simulink model "MassTransfer"  (R2023a)
settings: Solver=ode4  StartTime=0.0  StopTime=7540  FixedStep=Delta  RelTol=1e-3
values from neighbouring files (symbols this model uses):
  C2Ini = 1.6    [MassTransferModelData.m]
  C3Ini = 0    [MassTransferModelData.m]
  C4Ini = 0    [MassTransferModelData.m]
  C5Ini = 1.6    [MassTransferModelData.m]
  Delta = 5    [MassTransferModelData.m]
  F = 96485    [MassTransferModelData.m]
  NCells = 120    [MassTransferModelData.m]
  VCell = 0.4968    [MassTransferModelData.m]
  VTank = 500    [MassTransferModelData.m]
  z = 1    [MassTransferModelData.m]
undefined symbols (not defined in the file or in its folder): DiscIntNeverNeededParam
(part 1 of 3)
settings Model: Creator=801896  LastModifiedBy=801896

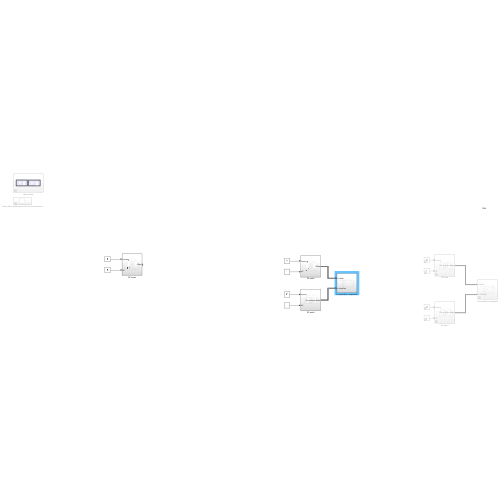
[thumbnail: Simulink's stored preview of the top-level diagram]
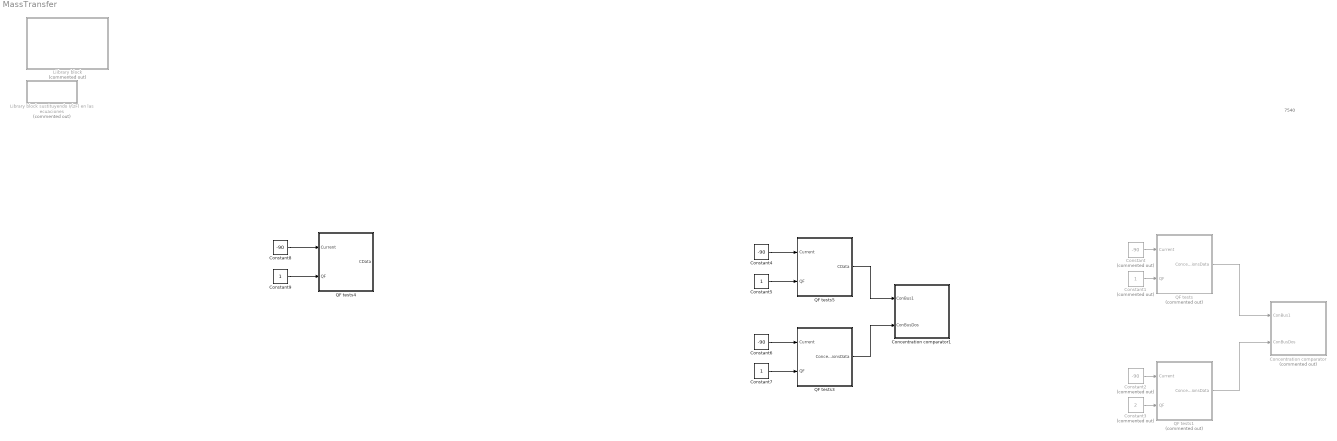
== system MassTransfer ==
  note: 7540
  Concentration comparator : Subsystem  Commented=on
  Concentration comparator1 : Subsystem
  Constant : Constant  Commented=on  Value=-90
  Constant1 : Constant  Commented=on
  Constant2 : Constant  Commented=on  Value=-90
  Constant3 : Constant  Commented=on  Value=2
  Constant4 : Constant  Value=-90
  Constant5 : Constant
  Constant6 : Constant  Value=-90
  Constant7 : Constant
  Constant8 : Constant  Value=-90
  Constant9 : Constant
  Library block sustituyendo I/(zF) en las ecuaciones : Subsystem  Commented=on
  Liibrary block : Subsystem  Commented=on
  QF tests : Subsystem  Commented=on
  QF tests1 : Subsystem  Commented=on
  QF tests3 : Subsystem
  QF tests4 : Subsystem
  QF tests5 : Subsystem
  wires:
  Constant/1 -> QF tests/1(Current)
  Constant1/1 -> QF tests/2(QF)
  Constant2/1 -> QF tests1/1(Current)
  Constant3/1 -> QF tests1/2(QF)
  QF tests/1(ConcentrationsData) -> Concentration comparator/1(ConBus1)
  QF tests1/1(ConcentrationsData) -> Concentration comparator/2(ConBusDos)
  Constant4/1 -> QF tests5/1(Current)
  Constant5/1 -> QF tests5/2(QF)
  Constant6/1 -> QF tests3/1(Current)
  Constant7/1 -> QF tests3/2(QF)
  QF tests5/1(CData) -> Concentration comparator1/1(ConBus1)
  QF tests3/1(ConcentrationsData) -> Concentration comparator1/2(ConBusDos)
  Constant8/1 -> QF tests4/1(Current)
  Constant9/1 -> QF tests4/2(QF)

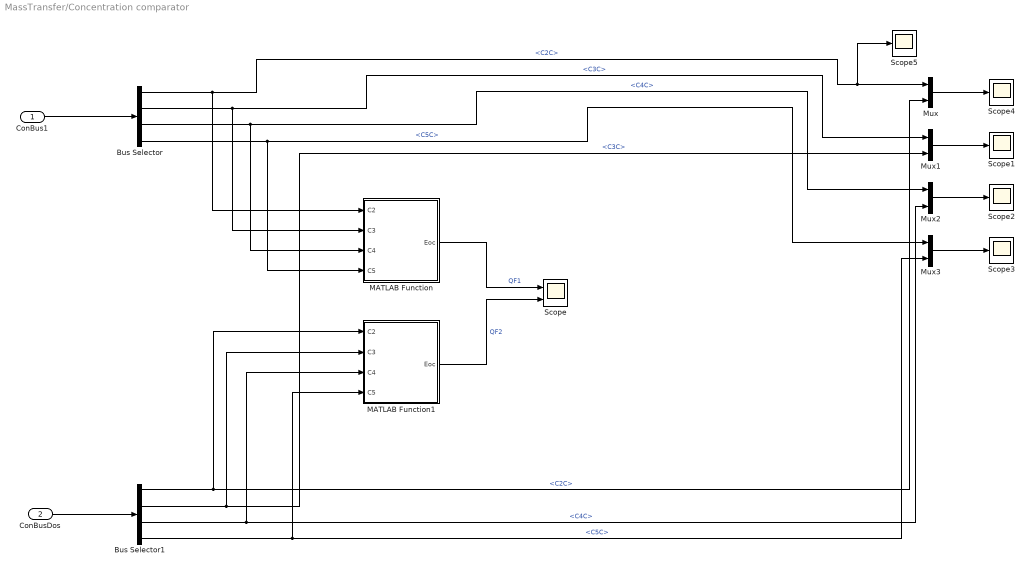
== system MassTransfer/Concentration comparator ==
  ConBus1 : Inport
  ConBusDos : Inport  Port=2
  Bus Selector : BusSelector  OutputSignals=C2C,C3C,C4C,C5C
  Bus Selector1 : BusSelector  OutputSignals=C2C,C3C,C4C,C5C
  MATLAB Function : MATLAB Function  TreatAsAtomicUnit=on
  MATLAB Function1 : MATLAB Function  TreatAsAtomicUnit=on
  Mux{,1..3} (4 alike) : Mux  Inputs=2
  Scope : Scope  NumInputPorts=2
  Scope{1..5} (5 alike) : Scope
  wires:
  ConBus1/1 -> Bus Selector/1
  ConBusDos/1 -> Bus Selector1/1
  Bus Selector/1 -> MATLAB Function/1(C2), Scope5/1, Mux/1  "<C2C>"
  Bus Selector1/1 -> MATLAB Function1/1(C2), Mux/2  "<C2C>"
  Bus Selector/2 -> MATLAB Function/2(C3), Mux1/1  "<C3C>"
  Bus Selector1/2 -> MATLAB Function1/2(C3), Mux1/2  "<C3C>"
  Bus Selector/3 -> MATLAB Function/3(C4), Mux2/1  "<C4C>"
  Bus Selector1/3 -> MATLAB Function1/3(C4), Mux2/2  "<C4C>"
  Bus Selector1/4 -> MATLAB Function1/4(C5), Mux3/2  "<C5C>"
  Bus Selector/4 -> MATLAB Function/4(C5), Mux3/1  "<C5C>"
  Mux1/1 -> Scope1/1
  Mux2/1 -> Scope2/1
  Mux3/1 -> Scope3/1
  Mux/1 -> Scope4/1
  MATLAB Function/1(Eoc) -> Scope/1  "QF1"
  MATLAB Function1/1(Eoc) -> Scope/2  "QF2"

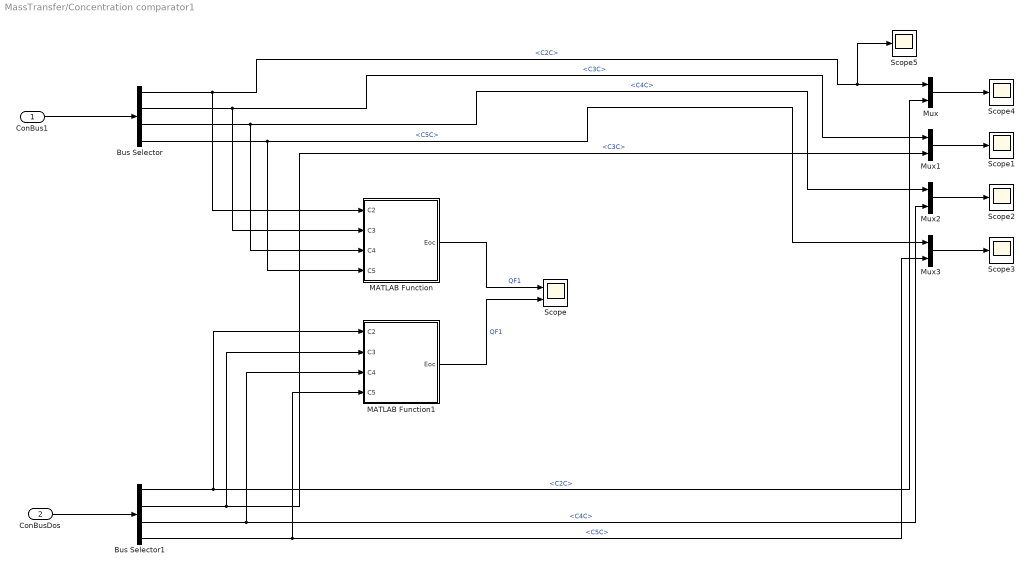
== system MassTransfer/Concentration comparator1 ==
  ConBus1 : Inport
  ConBusDos : Inport  Port=2
  Bus Selector : BusSelector  OutputSignals=C2C,C3C,C4C,C5C
  Bus Selector1 : BusSelector  OutputSignals=C2C,C3C,C4C,C5C
  MATLAB Function : MATLAB Function  TreatAsAtomicUnit=on
  MATLAB Function1 : MATLAB Function  TreatAsAtomicUnit=on
  Mux{,1..3} (4 alike) : Mux  Inputs=2
  Scope : Scope  NumInputPorts=2
  Scope{1..5} (5 alike) : Scope
  wires:
  MATLAB Function1/1(Eoc) -> Scope/2  "QF1"
  MATLAB Function/1(Eoc) -> Scope/1  "QF1"
  Mux/1 -> Scope4/1
  Mux3/1 -> Scope3/1
  Mux2/1 -> Scope2/1
  Mux1/1 -> Scope1/1
  Bus Selector/4 -> Mux3/1, MATLAB Function/4(C5)  "<C5C>"
  Bus Selector1/4 -> Mux3/2, MATLAB Function1/4(C5)  "<C5C>"
  Bus Selector1/3 -> Mux2/2, MATLAB Function1/3(C4)  "<C4C>"
  Bus Selector/3 -> Mux2/1, MATLAB Function/3(C4)  "<C4C>"
  Bus Selector1/2 -> Mux1/2, MATLAB Function1/2(C3)  "<C3C>"
  Bus Selector/2 -> Mux1/1, MATLAB Function/2(C3)  "<C3C>"
  Bus Selector1/1 -> Mux/2, MATLAB Function1/1(C2)  "<C2C>"
  Bus Selector/1 -> Mux/1, Scope5/1, MATLAB Function/1(C2)  "<C2C>"
  ConBusDos/1 -> Bus Selector1/1
  ConBus1/1 -> Bus Selector/1

== system MassTransfer/Library block sustituyendo I//(zF) en las ecuaciones ==
  QF tests2 : Subsystem

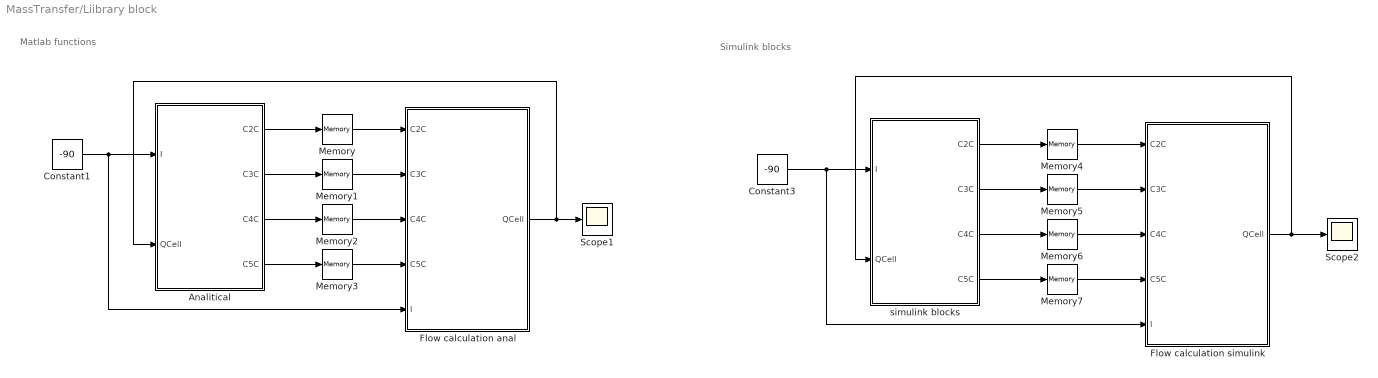
== system MassTransfer/Liibrary block ==
  note: Matlab functions
  note: Simulink blocks
  Analitical : Subsystem
  Constant1 : Constant  Value=-90
  Constant3 : Constant  Value=-90
  Flow calculation anal : Subsystem
  Flow calculation simulink : Subsystem
  Memory : Memory  InitialCondition=C2Ini
  Memory1 : Memory  InitialCondition=C3Ini
  Memory2 : Memory  InitialCondition=C4Ini
  Memory3 : Memory  InitialCondition=C5Ini
  Memory4 : Memory  InitialCondition=C2Ini
  Memory5 : Memory  InitialCondition=C3Ini
  Memory6 : Memory  InitialCondition=C4Ini
  Memory7 : Memory  InitialCondition=C5Ini
  Scope1 : Scope
  Scope2 : Scope
  simulink blocks : Subsystem
  wires:
  Memory4/1 -> Flow calculation simulink/1(C2C)
  Memory6/1 -> Flow calculation simulink/3(C4C)
  Flow calculation simulink/1(QCell) -> Scope2/1, simulink blocks/2(QCell)
  Constant3/1 -> Flow calculation simulink/5(I), simulink blocks/1(I)
  Memory7/1 -> Flow calculation simulink/4(C5C)
  Memory5/1 -> Flow calculation simulink/2(C3C)
  simulink blocks/2(C3C) -> Memory5/1
  simulink blocks/1(C2C) -> Memory4/1
  Analitical/4(C5C) -> Memory3/1
  Analitical/2(C3C) -> Memory1/1
  simulink blocks/4(C5C) -> Memory7/1
  Constant1/1 -> Flow calculation anal/5(I), Analitical/1(I)
  Memory/1 -> Flow calculation anal/1(C2C)
  Analitical/1(C2C) -> Memory/1
  Memory2/1 -> Flow calculation anal/3(C4C)
  Flow calculation anal/1(QCell) -> Analitical/2(QCell), Scope1/1
  Memory3/1 -> Flow calculation anal/4(C5C)
  Memory1/1 -> Flow calculation anal/2(C3C)
  Analitical/3(C4C) -> Memory2/1
  simulink blocks/3(C4C) -> Memory6/1

== system MassTransfer/QF tests ==
  Current : Inport
  QF : Inport  Port=2
  Analitical : Subsystem
  Flow calculation anal : Subsystem
      settings: PortSchema="{\"entries\":[{\"content\":{\"sides\":[{\"content\":{\"connectorIds\":[\"In1\",\"In2\",\"In3\",\"In4\",\"In5\"]},\"type\":\"ConnectorPlacement.EquallySpacedRectSide\",\"uuid\":\"0a7af6ce-45ad-4d0d-857c-093bf21aa09d\"},{\"content\":{\"connectorIds\":[\"Out1\"],\"side\":\"RIGHT\"},\"type\":\"ConnectorPlacement.EquallySpacedRectSide\",\"uuid\":\"931552ee-56bb-4ad6-a61d-ba39909d27e2\"},{\"content\":{\"side\":\"TOP\"},\"type\":\"ConnectorPlacement.EquallySpacedRectSide\",\"uuid\":\"a7ae0aa1-b7b5-4b34-b024-db37edb6a1ff\"},{\"content\":{\"connectorIds\":[\"In6\"],\"side\":\"BOTTOM\"},\"type\":\"ConnectorPlacement.EquallySpacedRectSide\",\"uuid\":\"41f7f592-25bc-4c7a-a534-5b1f71ad0dff\"}]},\"type\":\"ConnectorPlacement.EquallySpacedConnector\",\"uuid\":\"299fbe74-f349-4e94-b2aa-b85dedfa89e2\"}],\"packageUris\":[\"http://schema.mathworks.com/mf0/Connector/R2020b\"],\"version\":\"1.0\"}"
  Memory : Memory  InitialCondition=C2Ini
  Memory1 : Memory  InitialCondition=C3Ini
  Memory2 : Memory  InitialCondition=C4Ini
  Memory3 : Memory  InitialCondition=C5Ini
  Scope1 : Scope
  ConcentrationsData : Outport
  wires:
  Analitical/4(C5C) -> Memory3/1
  Analitical/2(C3C) -> Memory1/1
  Memory/1 -> Flow calculation anal/1(C2C)
  Analitical/1(C2C) -> Memory/1
  Memory2/1 -> Flow calculation anal/3(C4C)
  Flow calculation anal/1(QCell) -> Analitical/2(QCell), Scope1/1
  Memory3/1 -> Flow calculation anal/4(C5C)
  Memory1/1 -> Flow calculation anal/2(C3C)
  Analitical/3(C4C) -> Memory2/1
  QF/1 -> Flow calculation anal/6(QF)
  Current/1 -> Flow calculation anal/5(I), Analitical/1(I)
  Analitical/5(ConcentrationsData) -> ConcentrationsData/1

== system MassTransfer/QF tests1 ==
  Current : Inport
  QF : Inport  Port=2
  Analitical : Subsystem
  Flow calculation anal : Subsystem
      settings: PortSchema="{\"entries\":[{\"content\":{\"sides\":[{\"content\":{\"connectorIds\":[\"In1\",\"In2\",\"In3\",\"In4\",\"In5\"]},\"type\":\"ConnectorPlacement.EquallySpacedRectSide\",\"uuid\":\"0a7af6ce-45ad-4d0d-857c-093bf21aa09d\"},{\"content\":{\"connectorIds\":[\"Out1\"],\"side\":\"RIGHT\"},\"type\":\"ConnectorPlacement.EquallySpacedRectSide\",\"uuid\":\"931552ee-56bb-4ad6-a61d-ba39909d27e2\"},{\"content\":{\"side\":\"TOP\"},\"type\":\"ConnectorPlacement.EquallySpacedRectSide\",\"uuid\":\"a7ae0aa1-b7b5-4b34-b024-db37edb6a1ff\"},{\"content\":{\"connectorIds\":[\"In6\"],\"side\":\"BOTTOM\"},\"type\":\"ConnectorPlacement.EquallySpacedRectSide\",\"uuid\":\"41f7f592-25bc-4c7a-a534-5b1f71ad0dff\"}]},\"type\":\"ConnectorPlacement.EquallySpacedConnector\",\"uuid\":\"299fbe74-f349-4e94-b2aa-b85dedfa89e2\"}],\"packageUris\":[\"http://schema.mathworks.com/mf0/Connector/R2020b\"],\"version\":\"1.0\"}"
  Memory : Memory  InitialCondition=C2Ini
  Memory1 : Memory  InitialCondition=C3Ini
  Memory2 : Memory  InitialCondition=C4Ini
  Memory3 : Memory  InitialCondition=C5Ini
  Scope1 : Scope
  ConcentrationsData : Outport
  wires:
  Analitical/5(ConcentrationsData) -> ConcentrationsData/1
  Current/1 -> Analitical/1(I), Flow calculation anal/5(I)
  QF/1 -> Flow calculation anal/6(QF)
  Analitical/3(C4C) -> Memory2/1
  Memory1/1 -> Flow calculation anal/2(C3C)
  Memory3/1 -> Flow calculation anal/4(C5C)
  Flow calculation anal/1(QCell) -> Scope1/1, Analitical/2(QCell)
  Memory2/1 -> Flow calculation anal/3(C4C)
  Analitical/1(C2C) -> Memory/1
  Memory/1 -> Flow calculation anal/1(C2C)
  Analitical/2(C3C) -> Memory1/1
  Analitical/4(C5C) -> Memory3/1

== system MassTransfer/QF tests3 ==
  Current : Inport
  QF : Inport  Port=2
  Analitical : Subsystem
  Flow calculation anal : Subsystem
      settings: PortSchema="{\"entries\":[{\"content\":{\"sides\":[{\"content\":{\"connectorIds\":[\"In1\",\"In2\",\"In3\",\"In4\",\"In5\"]},\"type\":\"ConnectorPlacement.EquallySpacedRectSide\",\"uuid\":\"0a7af6ce-45ad-4d0d-857c-093bf21aa09d\"},{\"content\":{\"connectorIds\":[\"Out1\"],\"side\":\"RIGHT\"},\"type\":\"ConnectorPlacement.EquallySpacedRectSide\",\"uuid\":\"931552ee-56bb-4ad6-a61d-ba39909d27e2\"},{\"content\":{\"side\":\"TOP\"},\"type\":\"ConnectorPlacement.EquallySpacedRectSide\",\"uuid\":\"a7ae0aa1-b7b5-4b34-b024-db37edb6a1ff\"},{\"content\":{\"connectorIds\":[\"In6\"],\"side\":\"BOTTOM\"},\"type\":\"ConnectorPlacement.EquallySpacedRectSide\",\"uuid\":\"41f7f592-25bc-4c7a-a534-5b1f71ad0dff\"}]},\"type\":\"ConnectorPlacement.EquallySpacedConnector\",\"uuid\":\"299fbe74-f349-4e94-b2aa-b85dedfa89e2\"}],\"packageUris\":[\"http://schema.mathworks.com/mf0/Connector/R2020b\"],\"version\":\"1.0\"}"
  Memory : Memory  InitialCondition=C2Ini
  Memory1 : Memory  InitialCondition=C3Ini
  Memory2 : Memory  InitialCondition=C4Ini
  Memory3 : Memory  InitialCondition=C5Ini
  Scope1 : Scope
  ConcentrationsData : Outport
  wires:
  Analitical/5(ConcentrationsData) -> ConcentrationsData/1
  Current/1 -> Analitical/1(I), Flow calculation anal/5(I)
  QF/1 -> Flow calculation anal/6(QF)
  Analitical/3(C4C) -> Memory2/1
  Memory1/1 -> Flow calculation anal/2(C3C)
  Memory3/1 -> Flow calculation anal/4(C5C)
  Flow calculation anal/1(QCell) -> Scope1/1, Analitical/2(QCell)
  Memory2/1 -> Flow calculation anal/3(C4C)
  Analitical/1(C2C) -> Memory/1
  Memory/1 -> Flow calculation anal/1(C2C)
  Analitical/2(C3C) -> Memory1/1
  Analitical/4(C5C) -> Memory3/1

== system MassTransfer/QF tests4 ==
  Current : Inport
  QF : Inport  Port=2
  " Sim " : Subsystem
      settings: PortSchema="{\"entries\":[{\"content\":{\"sides\":[{\"content\":{\"connectorIds\":[\"In1\"]},\"type\":\"ConnectorPlacement.EquallySpacedRectSide\",\"uuid\":\"0af2fe12-92e2-4934-8caf-d0e09156ac6e\"},{\"content\":{\"connectorIds\":[\"Out1\",\"Out2\",\"Out3\",\"Out4\"],\"side\":\"RIGHT\"},\"type\":\"ConnectorPlacement.EquallySpacedRectSide\",\"uuid\":\"b4f72661-341b-4f6c-9f31-b95dca80a872\"},{\"content\":{\"connectorIds\":[\"In2\"],\"side\":\"TOP\"},\"type\":\"ConnectorPlacement.EquallySpacedRectSide\",\"uuid\":\"c5190f73-027e-4f11-a56f-d8aaac8187a8\"},{\"content\":{\"connectorIds\":[\"In3\",\"Out5\"],\"side\":\"BOTTOM\"},\"type\":\"ConnectorPlacement.EquallySpacedRectSide\",\"uuid\":\"f82a3118-5f16-4772-b644-cc59a9b71989\"}]},\"type\":\"ConnectorPlacement.EquallySpacedConnector\",\"uuid\":\"9ff8b57e-c184-4695-a7f3-1246e68507a5\"}],\"packageUris\":[\"http://schema.mathworks.com/mf0/Connector/R2020b\"],\"version\":\"1.0\"}"
  Flow calculation anal : Subsystem
      settings: PortSchema="{\"entries\":[{\"content\":{\"sides\":[{\"content\":{\"connectorIds\":[\"In1\",\"In2\",\"In3\",\"In4\"]},\"type\":\"ConnectorPlacement.EquallySpacedRectSide\",\"uuid\":\"0a7af6ce-45ad-4d0d-857c-093bf21aa09d\"},{\"content\":{\"connectorIds\":[\"Out1\"],\"side\":\"RIGHT\"},\"type\":\"ConnectorPlacement.EquallySpacedRectSide\",\"uuid\":\"931552ee-56bb-4ad6-a61d-ba39909d27e2\"},{\"content\":{\"connectorIds\":[\"In5\"],\"side\":\"TOP\"},\"type\":\"ConnectorPlacement.EquallySpacedRectSide\",\"uuid\":\"a7ae0aa1-b7b5-4b34-b024-db37edb6a1ff\"},{\"content\":{\"connectorIds\":[\"In6\"],\"side\":\"BOTTOM\"},\"type\":\"ConnectorPlacement.EquallySpacedRectSide\",\"uuid\":\"41f7f592-25bc-4c7a-a534-5b1f71ad0dff\"}]},\"type\":\"ConnectorPlacement.EquallySpacedConnector\",\"uuid\":\"299fbe74-f349-4e94-b2aa-b85dedfa89e2\"}],\"packageUris\":[\"http://schema.mathworks.com/mf0/Connector/R2020b\"],\"version\":\"1.0\"}"
  Memory : Memory  InitialCondition=C2Ini
  Memory1 : Memory  InitialCondition=C3Ini
  Memory2 : Memory  InitialCondition=C4Ini
  Memory3 : Memory  InitialCondition=C5Ini
  Scope1 : Scope
  CData : Outport
  wires:
  " Sim "/3(C4C) -> Memory2/1
  Memory1/1 -> Flow calculation anal/2(C3C)
  Memory3/1 -> Flow calculation anal/4(C5C)
  Memory2/1 -> Flow calculation anal/3(C4C)
  " Sim "/1(C2C) -> Memory/1
  Memory/1 -> Flow calculation anal/1(C2C)
  " Sim "/2(C3C) -> Memory1/1
  " Sim "/4(C5C) -> Memory3/1
  QF/1 -> Flow calculation anal/5(QF), " Sim "/2(QF)
  Flow calculation anal/1(QCell) -> Scope1/1, " Sim "/1(QCell)
  Current/1 -> Flow calculation anal/6(I), " Sim "/3(I)
  " Sim "/5(ConcentrationsData) -> CData/1

== system MassTransfer/QF tests5 ==
  Current : Inport
  QF : Inport  Port=2
  " Sim " : Subsystem
      settings: PortSchema="{\"entries\":[{\"content\":{\"sides\":[{\"content\":{\"connectorIds\":[\"In1\"]},\"type\":\"ConnectorPlacement.EquallySpacedRectSide\",\"uuid\":\"0af2fe12-92e2-4934-8caf-d0e09156ac6e\"},{\"content\":{\"connectorIds\":[\"Out1\",\"Out2\",\"Out3\",\"Out4\"],\"side\":\"RIGHT\"},\"type\":\"ConnectorPlacement.EquallySpacedRectSide\",\"uuid\":\"b4f72661-341b-4f6c-9f31-b95dca80a872\"},{\"content\":{\"connectorIds\":[\"In2\"],\"side\":\"TOP\"},\"type\":\"ConnectorPlacement.EquallySpacedRectSide\",\"uuid\":\"c5190f73-027e-4f11-a56f-d8aaac8187a8\"},{\"content\":{\"connectorIds\":[\"In3\",\"Out5\"],\"side\":\"BOTTOM\"},\"type\":\"ConnectorPlacement.EquallySpacedRectSide\",\"uuid\":\"f82a3118-5f16-4772-b644-cc59a9b71989\"}]},\"type\":\"ConnectorPlacement.EquallySpacedConnector\",\"uuid\":\"9ff8b57e-c184-4695-a7f3-1246e68507a5\"}],\"packageUris\":[\"http://schema.mathworks.com/mf0/Connector/R2020b\"],\"version\":\"1.0\"}"
  Flow calculation anal : Subsystem
      settings: PortSchema="{\"entries\":[{\"content\":{\"sides\":[{\"content\":{\"connectorIds\":[\"In1\",\"In2\",\"In3\",\"In4\"]},\"type\":\"ConnectorPlacement.EquallySpacedRectSide\",\"uuid\":\"0a7af6ce-45ad-4d0d-857c-093bf21aa09d\"},{\"content\":{\"connectorIds\":[\"Out1\"],\"side\":\"RIGHT\"},\"type\":\"ConnectorPlacement.EquallySpacedRectSide\",\"uuid\":\"931552ee-56bb-4ad6-a61d-ba39909d27e2\"},{\"content\":{\"connectorIds\":[\"In5\"],\"side\":\"TOP\"},\"type\":\"ConnectorPlacement.EquallySpacedRectSide\",\"uuid\":\"a7ae0aa1-b7b5-4b34-b024-db37edb6a1ff\"},{\"content\":{\"connectorIds\":[\"In6\"],\"side\":\"BOTTOM\"},\"type\":\"ConnectorPlacement.EquallySpacedRectSide\",\"uuid\":\"41f7f592-25bc-4c7a-a534-5b1f71ad0dff\"}]},\"type\":\"ConnectorPlacement.EquallySpacedConnector\",\"uuid\":\"299fbe74-f349-4e94-b2aa-b85dedfa89e2\"}],\"packageUris\":[\"http://schema.mathworks.com/mf0/Connector/R2020b\"],\"version\":\"1.0\"}"
  Memory : Memory  InitialCondition=C2Ini
  Memory1 : Memory  InitialCondition=C3Ini
  Memory2 : Memory  InitialCondition=C4Ini
  Memory3 : Memory  InitialCondition=C5Ini
  Scope1 : Scope
  CData : Outport
  wires:
  " Sim "/5(ConcentrationsData) -> CData/1
  Current/1 -> " Sim "/3(I), Flow calculation anal/6(I)
  Flow calculation anal/1(QCell) -> " Sim "/1(QCell), Scope1/1
  QF/1 -> " Sim "/2(QF), Flow calculation anal/5(QF)
  " Sim "/4(C5C) -> Memory3/1
  " Sim "/2(C3C) -> Memory1/1
  Memory/1 -> Flow calculation anal/1(C2C)
  " Sim "/1(C2C) -> Memory/1
  Memory2/1 -> Flow calculation anal/3(C4C)
  Memory3/1 -> Flow calculation anal/4(C5C)
  Memory1/1 -> Flow calculation anal/2(C3C)
  " Sim "/3(C4C) -> Memory2/1

== system MassTransfer/Library block sustituyendo I//(zF) en las ecuaciones/QF tests2 ==
  Current : Inport
  QF : Inport  Port=2
  Flow calculation anal : Subsystem
      settings: PortSchema="{\"entries\":[{\"content\":{\"sides\":[{\"content\":{\"connectorIds\":[\"In1\",\"In2\",\"In3\",\"In4\",\"In5\"]},\"type\":\"ConnectorPlacement.EquallySpacedRectSide\",\"uuid\":\"0a7af6ce-45ad-4d0d-857c-093bf21aa09d\"},{\"content\":{\"connectorIds\":[\"Out1\"],\"side\":\"RIGHT\"},\"type\":\"ConnectorPlacement.EquallySpacedRectSide\",\"uuid\":\"931552ee-56bb-4ad6-a61d-ba39909d27e2\"},{\"content\":{\"side\":\"TOP\"},\"type\":\"ConnectorPlacement.EquallySpacedRectSide\",\"uuid\":\"a7ae0aa1-b7b5-4b34-b024-db37edb6a1ff\"},{\"content\":{\"connectorIds\":[\"In6\"],\"side\":\"BOTTOM\"},\"type\":\"ConnectorPlacement.EquallySpacedRectSide\",\"uuid\":\"41f7f592-25bc-4c7a-a534-5b1f71ad0dff\"}]},\"type\":\"ConnectorPlacement.EquallySpacedConnector\",\"uuid\":\"299fbe74-f349-4e94-b2aa-b85dedfa89e2\"}],\"packageUris\":[\"http://schema.mathworks.com/mf0/Connector/R2020b\"],\"version\":\"1.0\"}"
  Memory : Memory  InitialCondition=C2Ini
  Memory1 : Memory  InitialCondition=C3Ini
  Memory2 : Memory  InitialCondition=C4Ini
  Memory3 : Memory  InitialCondition=C5Ini
  Scope1 : Scope
  Simulink I/(zf) Cambiado : Subsystem
  ConcentrationsData : Outport
  wires:
  Simulink I/(zf) Cambiado/4(C5C) -> Memory3/1
  Simulink I/(zf) Cambiado/2(C3C) -> Memory1/1
  Memory/1 -> Flow calculation anal/1(C2C)
  Simulink I/(zf) Cambiado/1(C2C) -> Memory/1
  Memory2/1 -> Flow calculation anal/3(C4C)
  Flow calculation anal/1(QCell) -> Simulink I/(zf) Cambiado/2(QCell), Scope1/1
  Memory3/1 -> Flow calculation anal/4(C5C)
  Memory1/1 -> Flow calculation anal/2(C3C)
  Simulink I/(zf) Cambiado/3(C4C) -> Memory2/1
  QF/1 -> Simulink I/(zf) Cambiado/3(Qf), Flow calculation anal/6(QF)
  Current/1 -> Flow calculation anal/5(I), Simulink I/(zf) Cambiado/1(I)
  Simulink I/(zf) Cambiado/5(ConcentrationsData) -> ConcentrationsData/1

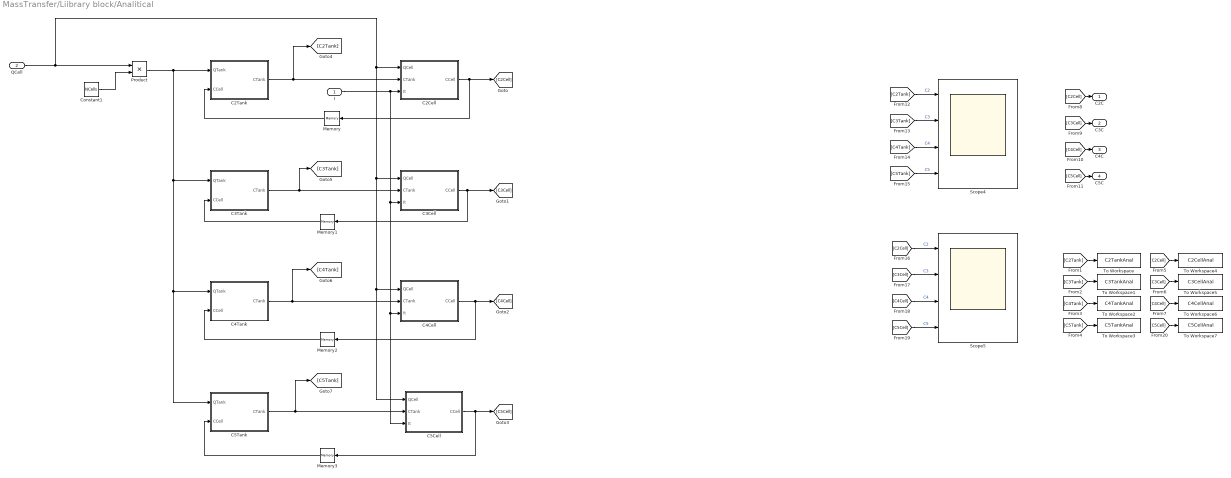
== system MassTransfer/Liibrary block/Analitical ==
  I : Inport
  QCell : Inport  Port=2
  C2Cell : Subsystem
  C2Tank : Subsystem
  C3Cell : Subsystem
  C3Tank : Subsystem
  C4Cell : Subsystem
  C4Tank : Subsystem
  C5Cell : Subsystem
  C5Tank : Subsystem
  Constant1 : Constant  Value=NCells
  Memory : Memory  InitialCondition=C2Ini
  Memory1 : Memory  InitialCondition=C3Ini
  Memory2 : Memory  InitialCondition=C4Ini
  Memory3 : Memory  InitialCondition=C5Ini
  Product : Product
  Scope4 : Scope  NumInputPorts=4
  Scope5 : Scope  NumInputPorts=4
  To Workspace : ToWorkspace  VariableName=C2TankAnal  SaveFormat=Timeseries  SampleTime=-1
  To Workspace1 : ToWorkspace  VariableName=C3TankAnal  SaveFormat=Timeseries  SampleTime=-1
  To Workspace2 : ToWorkspace  VariableName=C4TankAnal  SaveFormat=Timeseries  SampleTime=-1
  To Workspace3 : ToWorkspace  VariableName=C5TankAnal  SaveFormat=Timeseries  SampleTime=-1
  To Workspace4 : ToWorkspace  VariableName=C2CellAnal  SaveFormat=Timeseries  SampleTime=-1
  To Workspace5 : ToWorkspace  VariableName=C3CellAnal  SaveFormat=Timeseries  SampleTime=-1
  To Workspace6 : ToWorkspace  VariableName=C4CellAnal  SaveFormat=Timeseries  SampleTime=-1
  To Workspace7 : ToWorkspace  VariableName=C5CellAnal  SaveFormat=Timeseries  SampleTime=-1
  C2C : Outport
  C3C : Outport  Port=2
  C4C : Outport  Port=3
  C5C : Outport  Port=4
  wires:
  [C5Cell] -> C5C/1
  [C3Cell] -> C3C/1
  [C2Cell] -> C2C/1
  [C4Cell] -> C4C/1
  Constant1/1 -> Product/2
  QCell/1 -> C5Cell/1(QCell), C4Cell/1(QCell), C3Cell/1(QCell), C2Cell/1(QCell), Product/1
  C2Tank/1(CTank) -> [C2Tank], C2Cell/2(CTank)
  C2Cell/1(CCell) -> Memory/1, [C2Cell]
  C3Tank/1(CTank) -> [C3Tank], C3Cell/2(CTank)
  C3Cell/1(CCell) -> Memory1/1, [C3Cell]
  C5Tank/1(CTank) -> [C5Tank], C5Cell/2(CTank)
  C5Cell/1(CCell) -> Memory3/1, [C5Cell]
  C4Cell/1(CCell) -> Memory2/1, [C4Cell]
  C4Tank/1(CTank) -> [C4Tank], C4Cell/2(CTank)
  Product/1 -> C5Tank/1(QTank), C4Tank/1(QTank), C3Tank/1(QTank), C2Tank/1(QTank)
  I/1 -> C3Cell/3(It), C4Cell/3(It), C5Cell/3(It), C2Cell/3(It)
  Memory/1 -> C2Tank/2(CCell)
  Memory1/1 -> C3Tank/2(CCell)
  Memory2/1 -> C4Tank/2(CCell)
  Memory3/1 -> C5Tank/2(CCell)
  [C2Tank] -> Scope4/1  "C2"
  [C3Tank] -> Scope4/2  "C3"
  [C4Tank] -> Scope4/3  "C4"
  [C5Tank] -> Scope4/4  "C5"
  [C2Cell] -> Scope5/1  "C2"
  [C3Cell] -> Scope5/2  "C3"
  [C4Cell] -> Scope5/3  "C4"
  [C5Cell] -> Scope5/4  "C5"
  [C2Tank] -> To Workspace/1
  [C3Tank] -> To Workspace1/1
  [C4Tank] -> To Workspace2/1
  [C5Tank] -> To Workspace3/1
  [C2Cell] -> To Workspace4/1
  [C3Cell] -> To Workspace5/1
  [C4Cell] -> To Workspace6/1
  [C5Cell] -> To Workspace7/1

== system MassTransfer/Liibrary block/Flow calculation anal ==
  C2C : Inport
  C3C : Inport  Port=2
  C4C : Inport  Port=3
  C5C : Inport  Port=4
  I : Inport  Port=5
  Constant : Constant  Value=F
  MATLAB Function : MATLAB Function  TreatAsAtomicUnit=on
  To Workspace : ToWorkspace  VariableName=QCellAnal  SaveFormat=Timeseries  SampleTime=-1
  QCell : Outport
  wires:
  I/1 -> MATLAB Function/5(I)
  Constant/1 -> MATLAB Function/6(F)
  MATLAB Function/1(QCell) -> To Workspace/1, QCell/1
  C2C/1 -> MATLAB Function/1(C2)
  C3C/1 -> MATLAB Function/2(C3)
  C4C/1 -> MATLAB Function/3(C4)
  C5C/1 -> MATLAB Function/4(C5)

== system MassTransfer/Liibrary block/Flow calculation simulink ==
  C2C : Inport
  C3C : Inport  Port=2
  C4C : Inport  Port=3
  C5C : Inport  Port=4
  I : Inport  Port=5
  Constant : Constant  Value=F
  MATLAB Function : MATLAB Function  TreatAsAtomicUnit=on
  To Workspace : ToWorkspace  VariableName=QCellSim  SaveFormat=Timeseries  SampleTime=-1
  QCell : Outport
  wires:
  C5C/1 -> MATLAB Function/4(C5)
  C4C/1 -> MATLAB Function/3(C4)
  C3C/1 -> MATLAB Function/2(C3)
  C2C/1 -> MATLAB Function/1(C2)
  MATLAB Function/1(QCell) -> To Workspace/1, QCell/1
  Constant/1 -> MATLAB Function/6(F)
  I/1 -> MATLAB Function/5(I)

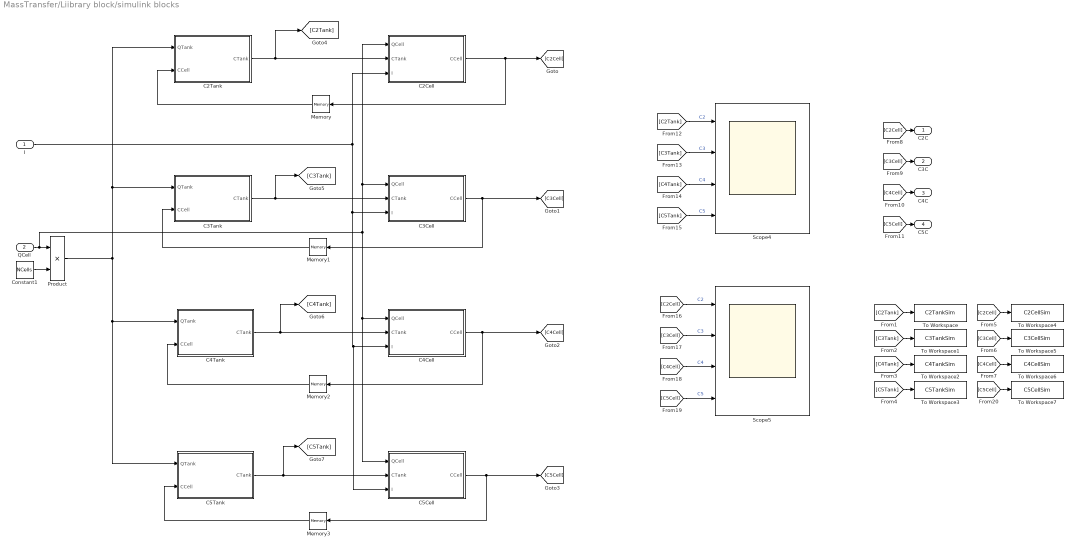
== system MassTransfer/Liibrary block/simulink blocks ==
  I : Inport
  QCell : Inport  Port=2
  C2Cell : Subsystem
  C2Tank : Subsystem
  C3Cell : Subsystem
  C3Tank : Subsystem
  C4Cell : Subsystem
  C4Tank : Subsystem
  C5Cell : Subsystem
  C5Tank : Subsystem
  Constant1 : Constant  Value=NCells
  Memory : Memory  InitialCondition=C2Ini
  Memory1 : Memory  InitialCondition=C3Ini
  Memory2 : Memory  InitialCondition=C4Ini
  Memory3 : Memory  InitialCondition=C5Ini
  Product : Product
  Scope4 : Scope  NumInputPorts=4
  Scope5 : Scope  NumInputPorts=4
  To Workspace : ToWorkspace  VariableName=C2TankSim  SaveFormat=Timeseries  SampleTime=-1
  To Workspace1 : ToWorkspace  VariableName=C3TankSim  SaveFormat=Timeseries  SampleTime=-1
  To Workspace2 : ToWorkspace  VariableName=C4TankSim  SaveFormat=Timeseries  SampleTime=-1
  To Workspace3 : ToWorkspace  VariableName=C5TankSim  SaveFormat=Timeseries  SampleTime=-1
  To Workspace4 : ToWorkspace  VariableName=C2CellSim  SaveFormat=Timeseries  SampleTime=-1
  To Workspace5 : ToWorkspace  VariableName=C3CellSim  SaveFormat=Timeseries  SampleTime=-1
  To Workspace6 : ToWorkspace  VariableName=C4CellSim  SaveFormat=Timeseries  SampleTime=-1
  To Workspace7 : ToWorkspace  VariableName=C5CellSim  SaveFormat=Timeseries  SampleTime=-1
  C2C : Outport
  C3C : Outport  Port=2
  C4C : Outport  Port=3
  C5C : Outport  Port=4
  wires:
  Constant1/1 -> Product/2
  QCell/1 -> C2Cell/1(QCell), C3Cell/1(QCell), C5Cell/1(QCell), C4Cell/1(QCell), Product/1
  [C2Cell] -> C2C/1
  [C3Cell] -> C3C/1
  [C4Cell] -> C4C/1
  [C5Cell] -> C5C/1
  C5Tank/1(CTank) -> C5Cell/2(CTank), [C5Tank]
  C4Tank/1(CTank) -> [C4Tank], C4Cell/2(CTank)
  C3Tank/1(CTank) -> [C3Tank], C3Cell/2(CTank)
  C2Tank/1(CTank) -> [C2Tank], C2Cell/2(CTank)
  C2Cell/1(CCell) -> Memory/1, [C2Cell]
  C3Cell/1(CCell) -> [C3Cell], Memory1/1
  C4Cell/1(CCell) -> [C4Cell], Memory2/1
  C5Cell/1(CCell) -> [C5Cell], Memory3/1
  Memory1/1 -> C3Tank/2(CCell)
  Memory2/1 -> C4Tank/2(CCell)
  Memory3/1 -> C5Tank/2(CCell)
  Memory/1 -> C2Tank/2(CCell)
  Product/1 -> C4Tank/1(QTank), C5Tank/1(QTank), C3Tank/1(QTank), C2Tank/1(QTank)
  I/1 -> C2Cell/3(I), C5Cell/3(I), C4Cell/3(I), C3Cell/3(I)
  [C3Tank] -> Scope4/2  "C3"
  [C2Cell] -> Scope5/1  "C2"
  [C4Cell] -> Scope5/3  "C4"
  [C4Tank] -> Scope4/3  "C4"
  [C5Cell] -> Scope5/4  "C5"
  [C3Cell] -> Scope5/2  "C3"
  [C5Tank] -> Scope4/4  "C5"
  [C2Tank] -> Scope4/1  "C2"
  [C2Cell] -> To Workspace4/1
  [C5Cell] -> To Workspace7/1
  [C2Tank] -> To Workspace/1
  [C5Tank] -> To Workspace3/1
  [C3Tank] -> To Workspace1/1
  [C3Cell] -> To Workspace5/1
  [C4Cell] -> To Workspace6/1
  [C4Tank] -> To Workspace2/1

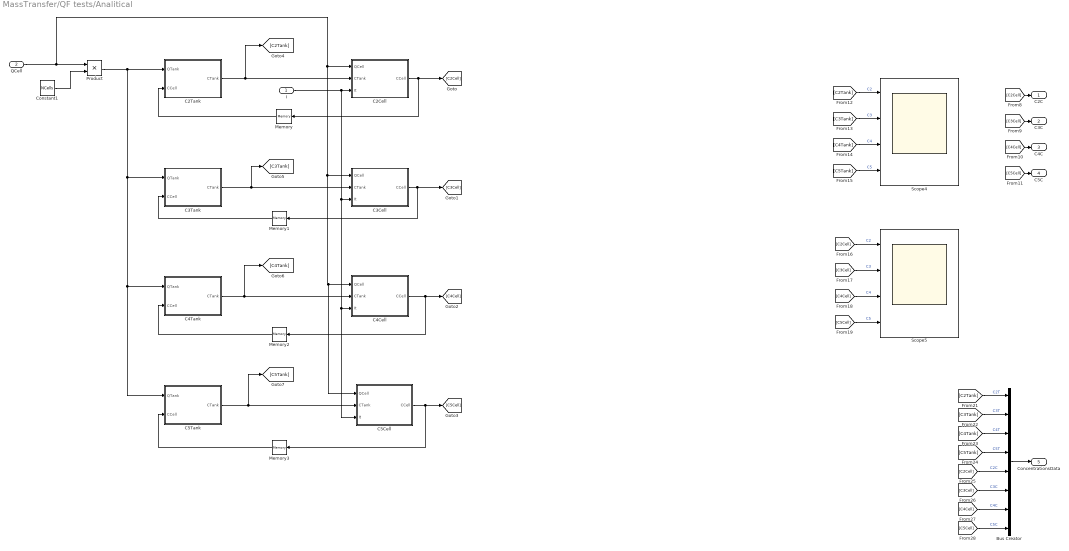
== system MassTransfer/QF tests/Analitical ==
  I : Inport
  QCell : Inport  Port=2
  Bus Creator : BusCreator  Inputs=8
  C2Cell : Subsystem
  C2Tank : Subsystem
  C3Cell : Subsystem
  C3Tank : Subsystem
  C4Cell : Subsystem
  C4Tank : Subsystem
  C5Cell : Subsystem
  C5Tank : Subsystem
  Constant1 : Constant  Value=NCells
  Memory : Memory  InitialCondition=C2Ini
  Memory1 : Memory  InitialCondition=C3Ini
  Memory2 : Memory  InitialCondition=C4Ini
  Memory3 : Memory  InitialCondition=C5Ini
  Product : Product
  Scope4 : Scope  NumInputPorts=4
  Scope5 : Scope  NumInputPorts=4
  C2C : Outport
  C3C : Outport  Port=2
  C4C : Outport  Port=3
  C5C : Outport  Port=4
  ConcentrationsData : Outport  Port=5
  wires:
  [C5Cell] -> C5C/1
  [C3Cell] -> C3C/1
  [C2Cell] -> C2C/1
  [C4Cell] -> C4C/1
  Constant1/1 -> Product/2
  QCell/1 -> C5Cell/1(QCell), C4Cell/1(QCell), C3Cell/1(QCell), C2Cell/1(QCell), Product/1
  C2Tank/1(CTank) -> [C2Tank], C2Cell/2(CTank)
  C2Cell/1(CCell) -> Memory/1, [C2Cell]
  C3Tank/1(CTank) -> [C3Tank], C3Cell/2(CTank)
  C3Cell/1(CCell) -> Memory1/1, [C3Cell]
  C5Tank/1(CTank) -> [C5Tank], C5Cell/2(CTank)
  C5Cell/1(CCell) -> Memory3/1, [C5Cell]
  C4Cell/1(CCell) -> Memory2/1, [C4Cell]
  C4Tank/1(CTank) -> [C4Tank], C4Cell/2(CTank)
  Product/1 -> C5Tank/1(QTank), C4Tank/1(QTank), C3Tank/1(QTank), C2Tank/1(QTank)
  I/1 -> C3Cell/3(It), C4Cell/3(It), C5Cell/3(It), C2Cell/3(It)
  Memory/1 -> C2Tank/2(CCell)
  Memory1/1 -> C3Tank/2(CCell)
  Memory2/1 -> C4Tank/2(CCell)
  Memory3/1 -> C5Tank/2(CCell)
  [C2Tank] -> Scope4/1  "C2"
  [C3Tank] -> Scope4/2  "C3"
  [C4Tank] -> Scope4/3  "C4"
  [C5Tank] -> Scope4/4  "C5"
  [C2Cell] -> Scope5/1  "C2"
  [C3Cell] -> Scope5/2  "C3"
  [C4Cell] -> Scope5/3  "C4"
  [C5Cell] -> Scope5/4  "C5"
  [C2Tank] -> Bus Creator/1  "C2T"
  [C3Tank] -> Bus Creator/2  "C3T"
  [C4Tank] -> Bus Creator/3  "C4T"
  [C5Tank] -> Bus Creator/4  "C5T"
  [C2Cell] -> Bus Creator/5  "C2C"
  [C3Cell] -> Bus Creator/6  "C3C"
  [C4Cell] -> Bus Creator/7  "C4C"
  [C5Cell] -> Bus Creator/8  "C5C"
  Bus Creator/1 -> ConcentrationsData/1

== system MassTransfer/QF tests/Flow calculation anal ==
  C2C : Inport
  C3C : Inport  Port=2
  C4C : Inport  Port=3
  C5C : Inport  Port=4
  I : Inport  Port=5
  QF : Inport  Port=6
  Constant : Constant  Value=F
  MATLAB Function : MATLAB Function  TreatAsAtomicUnit=on
  QCell : Outport
  wires:
  I/1 -> MATLAB Function/5(I)
  Constant/1 -> MATLAB Function/6(F)
  MATLAB Function/1(QCell) -> QCell/1
  C2C/1 -> MATLAB Function/1(C2)
  C3C/1 -> MATLAB Function/2(C3)
  C4C/1 -> MATLAB Function/3(C4)
  C5C/1 -> MATLAB Function/4(C5)
  QF/1 -> MATLAB Function/7(QF)

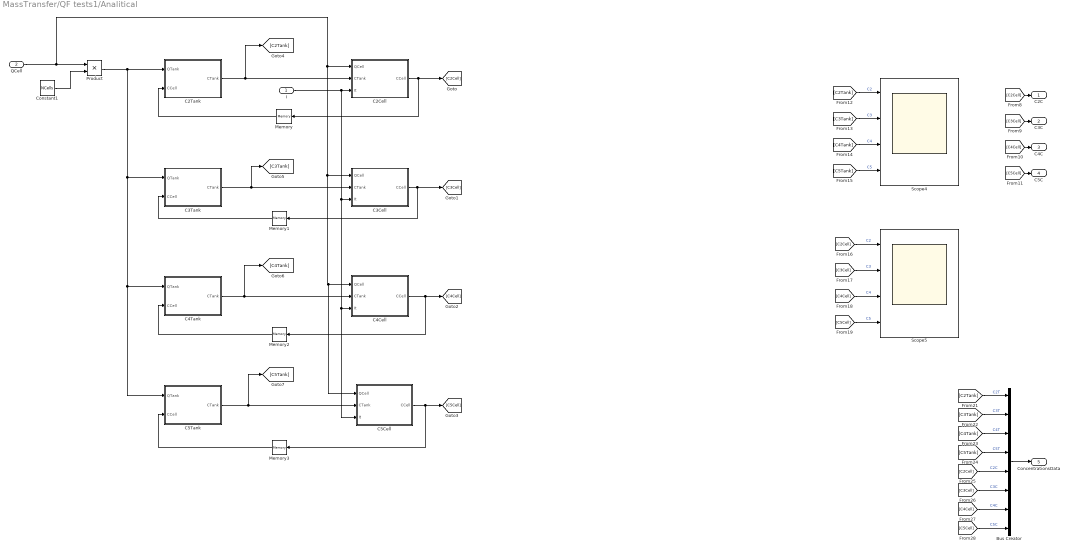
== system MassTransfer/QF tests1/Analitical ==
  I : Inport
  QCell : Inport  Port=2
  Bus Creator : BusCreator  Inputs=8
  C2Cell : Subsystem
  C2Tank : Subsystem
  C3Cell : Subsystem
  C3Tank : Subsystem
  C4Cell : Subsystem
  C4Tank : Subsystem
  C5Cell : Subsystem
  C5Tank : Subsystem
  Constant1 : Constant  Value=NCells
  Memory : Memory  InitialCondition=C2Ini
  Memory1 : Memory  InitialCondition=C3Ini
  Memory2 : Memory  InitialCondition=C4Ini
  Memory3 : Memory  InitialCondition=C5Ini
  Product : Product
  Scope4 : Scope  NumInputPorts=4
  Scope5 : Scope  NumInputPorts=4
  C2C : Outport
  C3C : Outport  Port=2
  C4C : Outport  Port=3
  C5C : Outport  Port=4
  ConcentrationsData : Outport  Port=5
  wires:
  Bus Creator/1 -> ConcentrationsData/1
  [C5Cell] -> Bus Creator/8  "C5C"
  [C4Cell] -> Bus Creator/7  "C4C"
  [C3Cell] -> Bus Creator/6  "C3C"
  [C2Cell] -> Bus Creator/5  "C2C"
  [C5Tank] -> Bus Creator/4  "C5T"
  [C4Tank] -> Bus Creator/3  "C4T"
  [C3Tank] -> Bus Creator/2  "C3T"
  [C2Tank] -> Bus Creator/1  "C2T"
  [C5Cell] -> Scope5/4  "C5"
  [C4Cell] -> Scope5/3  "C4"
  [C3Cell] -> Scope5/2  "C3"
  [C2Cell] -> Scope5/1  "C2"
  [C5Tank] -> Scope4/4  "C5"
  [C4Tank] -> Scope4/3  "C4"
  [C3Tank] -> Scope4/2  "C3"
  [C2Tank] -> Scope4/1  "C2"
  Memory3/1 -> C5Tank/2(CCell)
  Memory2/1 -> C4Tank/2(CCell)
  Memory1/1 -> C3Tank/2(CCell)
  Memory/1 -> C2Tank/2(CCell)
  I/1 -> C2Cell/3(It), C5Cell/3(It), C4Cell/3(It), C3Cell/3(It)
  Product/1 -> C2Tank/1(QTank), C3Tank/1(QTank), C4Tank/1(QTank), C5Tank/1(QTank)
  C4Tank/1(CTank) -> C4Cell/2(CTank), [C4Tank]
  C4Cell/1(CCell) -> [C4Cell], Memory2/1
  C5Cell/1(CCell) -> [C5Cell], Memory3/1
  C5Tank/1(CTank) -> C5Cell/2(CTank), [C5Tank]
  C3Cell/1(CCell) -> [C3Cell], Memory1/1
  C3Tank/1(CTank) -> C3Cell/2(CTank), [C3Tank]
  C2Cell/1(CCell) -> [C2Cell], Memory/1
  C2Tank/1(CTank) -> C2Cell/2(CTank), [C2Tank]
  QCell/1 -> Product/1, C2Cell/1(QCell), C3Cell/1(QCell), C4Cell/1(QCell), C5Cell/1(QCell)
  Constant1/1 -> Product/2
  [C4Cell] -> C4C/1
  [C2Cell] -> C2C/1
  [C3Cell] -> C3C/1
  [C5Cell] -> C5C/1

== system MassTransfer/QF tests1/Flow calculation anal ==
  C2C : Inport
  C3C : Inport  Port=2
  C4C : Inport  Port=3
  C5C : Inport  Port=4
  I : Inport  Port=5
  QF : Inport  Port=6
  Constant : Constant  Value=F
  MATLAB Function : MATLAB Function  TreatAsAtomicUnit=on
  QCell : Outport
  wires:
  QF/1 -> MATLAB Function/7(QF)
  C5C/1 -> MATLAB Function/4(C5)
  C4C/1 -> MATLAB Function/3(C4)
  C3C/1 -> MATLAB Function/2(C3)
  C2C/1 -> MATLAB Function/1(C2)
  MATLAB Function/1(QCell) -> QCell/1
  Constant/1 -> MATLAB Function/6(F)
  I/1 -> MATLAB Function/5(I)

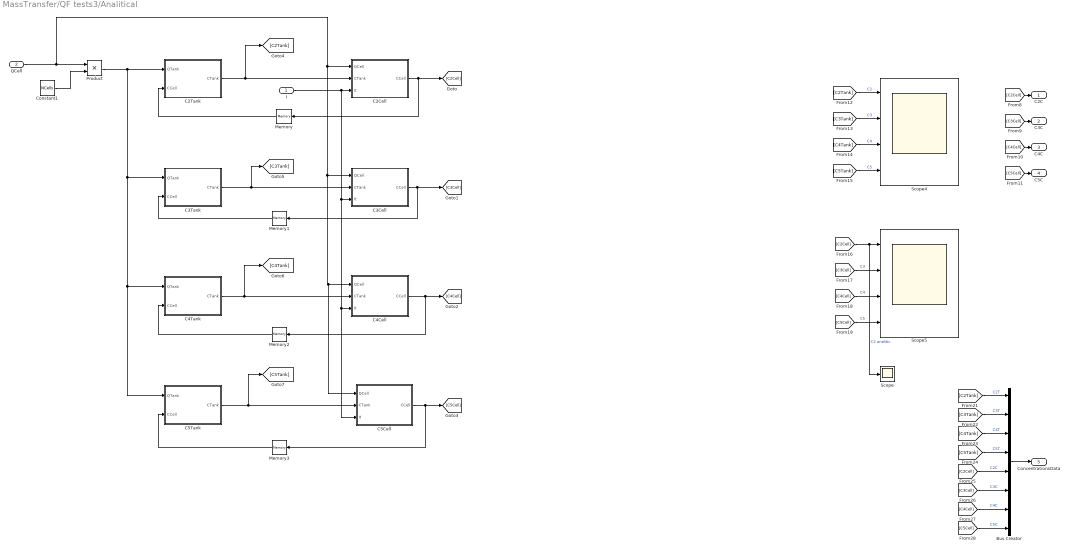
== system MassTransfer/QF tests3/Analitical ==
  I : Inport
  QCell : Inport  Port=2
  Bus Creator : BusCreator  Inputs=8
  C2Cell : Subsystem
  C2Tank : Subsystem
  C3Cell : Subsystem
  C3Tank : Subsystem
  C4Cell : Subsystem
  C4Tank : Subsystem
  C5Cell : Subsystem
  C5Tank : Subsystem
  Constant1 : Constant  Value=NCells
  Memory : Memory  InitialCondition=C2Ini
  Memory1 : Memory  InitialCondition=C3Ini
  Memory2 : Memory  InitialCondition=C4Ini
  Memory3 : Memory  InitialCondition=C5Ini
  Product : Product
  Scope : Scope
  Scope4 : Scope  NumInputPorts=4
  Scope5 : Scope  NumInputPorts=4
  C2C : Outport
  C3C : Outport  Port=2
  C4C : Outport  Port=3
  C5C : Outport  Port=4
  ConcentrationsData : Outport  Port=5
  wires:
  Bus Creator/1 -> ConcentrationsData/1
  [C5Cell] -> Bus Creator/8  "C5C"
  [C4Cell] -> Bus Creator/7  "C4C"
  [C3Cell] -> Bus Creator/6  "C3C"
  [C2Cell] -> Bus Creator/5  "C2C"
  [C5Tank] -> Bus Creator/4  "C5T"
  [C4Tank] -> Bus Creator/3  "C4T"
  [C3Tank] -> Bus Creator/2  "C3T"
  [C2Tank] -> Bus Creator/1  "C2T"
  [C5Cell] -> Scope5/4  "C5"
  [C4Cell] -> Scope5/3  "C4"
  [C3Cell] -> Scope5/2  "C3"
  [C2Cell] -> Scope/1, Scope5/1  "C2 analitic"
  [C5Tank] -> Scope4/4  "C5"
  [C4Tank] -> Scope4/3  "C4"
  [C3Tank] -> Scope4/2  "C3"
  [C2Tank] -> Scope4/1  "C2"
  Memory3/1 -> C5Tank/2(CCell)
  Memory2/1 -> C4Tank/2(CCell)
  Memory1/1 -> C3Tank/2(CCell)
  Memory/1 -> C2Tank/2(CCell)
  I/1 -> C2Cell/3(It), C5Cell/3(It), C4Cell/3(It), C3Cell/3(It)
  Product/1 -> C2Tank/1(QTank), C3Tank/1(QTank), C4Tank/1(QTank), C5Tank/1(QTank)
  C4Tank/1(CTank) -> C4Cell/2(CTank), [C4Tank]
  C4Cell/1(CCell) -> [C4Cell], Memory2/1
  C5Cell/1(CCell) -> [C5Cell], Memory3/1
  C5Tank/1(CTank) -> C5Cell/2(CTank), [C5Tank]
  C3Cell/1(CCell) -> [C3Cell], Memory1/1
  C3Tank/1(CTank) -> C3Cell/2(CTank), [C3Tank]
  C2Cell/1(CCell) -> [C2Cell], Memory/1
  C2Tank/1(CTank) -> C2Cell/2(CTank), [C2Tank]
  QCell/1 -> Product/1, C2Cell/1(QCell), C3Cell/1(QCell), C4Cell/1(QCell), C5Cell/1(QCell)
  Constant1/1 -> Product/2
  [C4Cell] -> C4C/1
  [C2Cell] -> C2C/1
  [C3Cell] -> C3C/1
  [C5Cell] -> C5C/1

== system MassTransfer/QF tests3/Flow calculation anal ==
  C2C : Inport
  C3C : Inport  Port=2
  C4C : Inport  Port=3
  C5C : Inport  Port=4
  I : Inport  Port=5
  QF : Inport  Port=6
  Constant : Constant  Value=F
  MATLAB Function : MATLAB Function  TreatAsAtomicUnit=on
  QCell : Outport
  wires:
  QF/1 -> MATLAB Function/7(QF)
  C5C/1 -> MATLAB Function/4(C5)
  C4C/1 -> MATLAB Function/3(C4)
  C3C/1 -> MATLAB Function/2(C3)
  C2C/1 -> MATLAB Function/1(C2)
  MATLAB Function/1(QCell) -> QCell/1
  Constant/1 -> MATLAB Function/6(F)
  I/1 -> MATLAB Function/5(I)

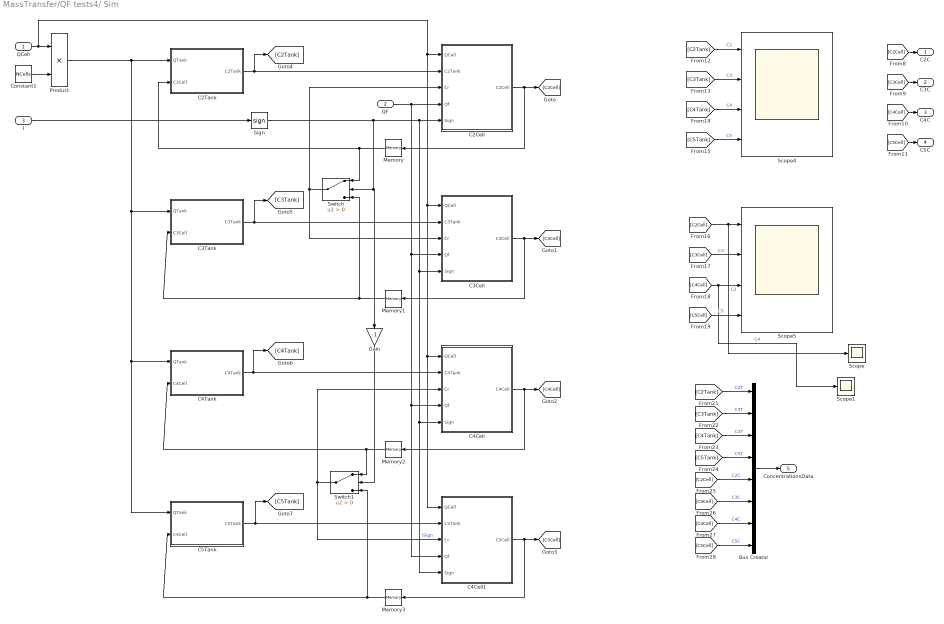
== system MassTransfer/QF tests4/ Sim  ==
  QCell : Inport
  QF : Inport  Port=2
  I : Inport  Port=3
  Bus Creator : BusCreator  Inputs=8
  C2Cell : Subsystem
  C2Tank : Subsystem
  C3Cell : Subsystem
  C3Tank : Subsystem
  C4Cell : Subsystem
  C4Cell1 : Subsystem
  C4Tank : Subsystem
  C5Tank : Subsystem
  Constant1 : Constant  Value=NCells
  Gain : Gain  Gain=-1
  Memory : Memory  InitialCondition=C2Ini
  Memory1 : Memory  InitialCondition=C3Ini
  Memory2 : Memory  InitialCondition=C4Ini
  Memory3 : Memory  InitialCondition=C5Ini
  Product : Product
  Scope : Scope
  Scope1 : Scope
  Scope4 : Scope  NumInputPorts=4
  Scope5 : Scope  NumInputPorts=4
  Sign : Signum
  Switch : Switch  Criteria=u2 > Threshold  SaturateOnIntegerOverflow=off  InputSameDT=off
  Switch1 : Switch  Criteria=u2 > Threshold  SaturateOnIntegerOverflow=off  InputSameDT=off
  C2C : Outport
  C3C : Outport  Port=2
  C4C : Outport  Port=3
  C5C : Outport  Port=4
  ConcentrationsData : Outport  Port=5
  wires:
  Gain/1 -> Switch1/2
  Switch1/1 -> C4Cell1/3(Cr), C4Cell/3(Cr)
  Switch/1 -> C2Cell/3(Cr), C3Cell/3(Cr)
  Product/1 -> C2Tank/1(QTank), C3Tank/1(QTank), C4Tank/1(QTank), C5Tank/1(QTank)
  Memory3/1 -> C5Tank/2(C5Cell), Switch1/3
  C4Cell1/1(C5Cell) -> Memory3/1, [C5Cell]
  Memory2/1 -> C4Tank/2(C4Cell), Switch1/1
  C4Cell/1(C4Cell) -> [C4Cell], Memory2/1
  Memory1/1 -> C3Tank/2(C3Cell), Switch/3
  C3Cell/1(C3Cell) -> [C3Cell], Memory1/1
  Memory/1 -> C2Tank/2(C2Cell), Switch/1
  C2Cell/1(C2Cell) -> [C2Cell], Memory/1
  C5Tank/1(C5Tank) -> C4Cell1/2(C5Tank), [C5Tank]
  C4Tank/1(C4Tank) -> C4Cell/2(C4Tank), [C4Tank]
  C3Tank/1(C3Tank) -> C3Cell/2(C3Tank), [C3Tank]
  C2Tank/1(C2Tank) -> [C2Tank], C2Cell/2(C2Tank)
  Sign/1 -> C2Cell/5(Sign), C4Cell/5(Sign), C4Cell1/5(Sign), C3Cell/5(Sign), Switch/2, Gain/1  "ISign"
  I/1 -> Sign/1
  QF/1 -> C2Cell/4(Qf), C4Cell/4(Qf), C4Cell1/4(Qf), C3Cell/4(Qf)
  Bus Creator/1 -> ConcentrationsData/1
  [C5Cell] -> Bus Creator/8  "C5C"
  [C4Cell] -> Bus Creator/7  "C4C"
  [C3Cell] -> Bus Creator/6  "C3C"
  [C2Cell] -> Bus Creator/5  "C2C"
  [C5Tank] -> Bus Creator/4  "C5T"
  [C4Tank] -> Bus Creator/3  "C4T"
  [C3Tank] -> Bus Creator/2  "C3T"
  [C2Tank] -> Bus Creator/1  "C2T"
  [C5Cell] -> Scope5/4  "C5"
  [C4Cell] -> Scope5/3, Scope1/1  "C4"
  [C3Cell] -> Scope5/2  "C3"
  [C2Cell] -> Scope5/1, Scope/1  "C2"
  [C5Tank] -> Scope4/4  "C5"
  [C4Tank] -> Scope4/3  "C4"
  [C3Tank] -> Scope4/2  "C3"
  [C2Tank] -> Scope4/1  "C2"
  QCell/1 -> Product/1, C3Cell/1(QCell), C4Cell/1(QCell), C4Cell1/1(QCell), C2Cell/1(QCell)
  Constant1/1 -> Product/2
  [C4Cell] -> C4C/1
  [C2Cell] -> C2C/1
  [C3Cell] -> C3C/1
  [C5Cell] -> C5C/1

== system MassTransfer/QF tests4/Flow calculation anal ==
  C2C : Inport
  C3C : Inport  Port=2
  C4C : Inport  Port=3
  C5C : Inport  Port=4
  QF : Inport  Port=5
  I : Inport  Port=6
  Constant : Constant  Value=F
  MATLAB Function : MATLAB Function  TreatAsAtomicUnit=on
  QCell : Outport
  wires:
  QF/1 -> MATLAB Function/7(QF)
  C5C/1 -> MATLAB Function/4(C5)
  C4C/1 -> MATLAB Function/3(C4)
  C3C/1 -> MATLAB Function/2(C3)
  C2C/1 -> MATLAB Function/1(C2)
  MATLAB Function/1(QCell) -> QCell/1
  Constant/1 -> MATLAB Function/6(F)
  I/1 -> MATLAB Function/5(I)

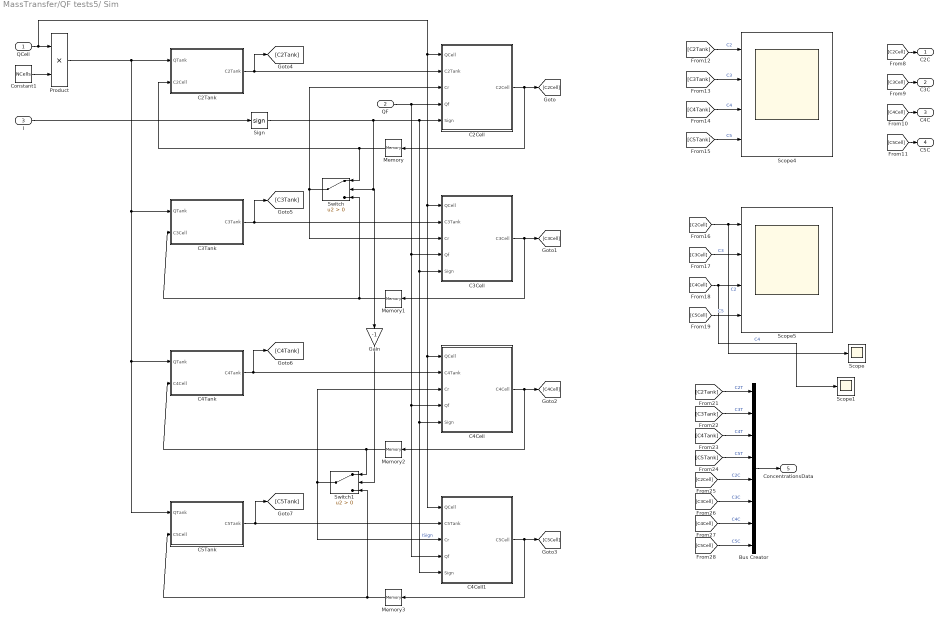
== system MassTransfer/QF tests5/ Sim  ==
  QCell : Inport
  QF : Inport  Port=2
  I : Inport  Port=3
  Bus Creator : BusCreator  Inputs=8
  C2Cell : Subsystem
  C2Tank : Subsystem
  C3Cell : Subsystem
  C3Tank : Subsystem
  C4Cell : Subsystem
  C4Cell1 : Subsystem
  C4Tank : Subsystem
  C5Tank : Subsystem
  Constant1 : Constant  Value=NCells
  Gain : Gain  Gain=-1
  Memory : Memory  InitialCondition=C2Ini
  Memory1 : Memory  InitialCondition=C3Ini
  Memory2 : Memory  InitialCondition=C4Ini
  Memory3 : Memory  InitialCondition=C5Ini
  Product : Product
  Scope : Scope
  Scope1 : Scope
  Scope4 : Scope  NumInputPorts=4
  Scope5 : Scope  NumInputPorts=4
  Sign : Signum
  Switch : Switch  Criteria=u2 > Threshold  SaturateOnIntegerOverflow=off  InputSameDT=off
  Switch1 : Switch  Criteria=u2 > Threshold  SaturateOnIntegerOverflow=off  InputSameDT=off
  C2C : Outport
  C3C : Outport  Port=2
  C4C : Outport  Port=3
  C5C : Outport  Port=4
  ConcentrationsData : Outport  Port=5
  wires:
  [C5Cell] -> C5C/1
  [C3Cell] -> C3C/1
  [C2Cell] -> C2C/1
  [C4Cell] -> C4C/1
  Constant1/1 -> Product/2
  QCell/1 -> C2Cell/1(QCell), C4Cell1/1(QCell), C4Cell/1(QCell), C3Cell/1(QCell), Product/1
  [C2Tank] -> Scope4/1  "C2"
  [C3Tank] -> Scope4/2  "C3"
  [C4Tank] -> Scope4/3  "C4"
  [C5Tank] -> Scope4/4  "C5"
  [C2Cell] -> Scope/1, Scope5/1  "C2"
  [C3Cell] -> Scope5/2  "C3"
  [C4Cell] -> Scope1/1, Scope5/3  "C4"
  [C5Cell] -> Scope5/4  "C5"
  [C2Tank] -> Bus Creator/1  "C2T"
  [C3Tank] -> Bus Creator/2  "C3T"
  [C4Tank] -> Bus Creator/3  "C4T"
  [C5Tank] -> Bus Creator/4  "C5T"
  [C2Cell] -> Bus Creator/5  "C2C"
  [C3Cell] -> Bus Creator/6  "C3C"
  [C4Cell] -> Bus Creator/7  "C4C"
  [C5Cell] -> Bus Creator/8  "C5C"
  Bus Creator/1 -> ConcentrationsData/1
  QF/1 -> C3Cell/4(Qf), C4Cell1/4(Qf), C4Cell/4(Qf), C2Cell/4(Qf)
  I/1 -> Sign/1
  Sign/1 -> Gain/1, Switch/2, C3Cell/5(Sign), C4Cell1/5(Sign), C4Cell/5(Sign), C2Cell/5(Sign)  "ISign"
  C2Tank/1(C2Tank) -> C2Cell/2(C2Tank), [C2Tank]
  C3Tank/1(C3Tank) -> [C3Tank], C3Cell/2(C3Tank)
  C4Tank/1(C4Tank) -> [C4Tank], C4Cell/2(C4Tank)
  C5Tank/1(C5Tank) -> [C5Tank], C4Cell1/2(C5Tank)
  C2Cell/1(C2Cell) -> Memory/1, [C2Cell]
  Memory/1 -> Switch/1, C2Tank/2(C2Cell)
  C3Cell/1(C3Cell) -> Memory1/1, [C3Cell]
  Memory1/1 -> Switch/3, C3Tank/2(C3Cell)
  C4Cell/1(C4Cell) -> Memory2/1, [C4Cell]
  Memory2/1 -> Switch1/1, C4Tank/2(C4Cell)
  C4Cell1/1(C5Cell) -> [C5Cell], Memory3/1
  Memory3/1 -> Switch1/3, C5Tank/2(C5Cell)
  Product/1 -> C5Tank/1(QTank), C4Tank/1(QTank), C3Tank/1(QTank), C2Tank/1(QTank)
  Switch/1 -> C3Cell/3(Cr), C2Cell/3(Cr)
  Switch1/1 -> C4Cell/3(Cr), C4Cell1/3(Cr)
  Gain/1 -> Switch1/2

== system MassTransfer/QF tests5/Flow calculation anal ==
  C2C : Inport
  C3C : Inport  Port=2
  C4C : Inport  Port=3
  C5C : Inport  Port=4
  QF : Inport  Port=5
  I : Inport  Port=6
  Constant : Constant  Value=F
  MATLAB Function : MATLAB Function  TreatAsAtomicUnit=on
  QCell : Outport
  wires:
  I/1 -> MATLAB Function/5(I)
  Constant/1 -> MATLAB Function/6(F)
  MATLAB Function/1(QCell) -> QCell/1
  C2C/1 -> MATLAB Function/1(C2)
  C3C/1 -> MATLAB Function/2(C3)
  C4C/1 -> MATLAB Function/3(C4)
  C5C/1 -> MATLAB Function/4(C5)
  QF/1 -> MATLAB Function/7(QF)

== system MassTransfer/Library block sustituyendo I//(zF) en las ecuaciones/QF tests2/Flow calculation anal ==
  C2C : Inport
  C3C : Inport  Port=2
  C4C : Inport  Port=3
  C5C : Inport  Port=4
  I : Inport  Port=5
  QF : Inport  Port=6
  Constant : Constant  Value=F
  MATLAB Function : MATLAB Function  TreatAsAtomicUnit=on
  QCell : Outport
  wires:
  I/1 -> MATLAB Function/5(I)
  Constant/1 -> MATLAB Function/6(F)
  MATLAB Function/1(QCell) -> QCell/1
  C2C/1 -> MATLAB Function/1(C2)
  C3C/1 -> MATLAB Function/2(C3)
  C4C/1 -> MATLAB Function/3(C4)
  C5C/1 -> MATLAB Function/4(C5)
  QF/1 -> MATLAB Function/7(QF)

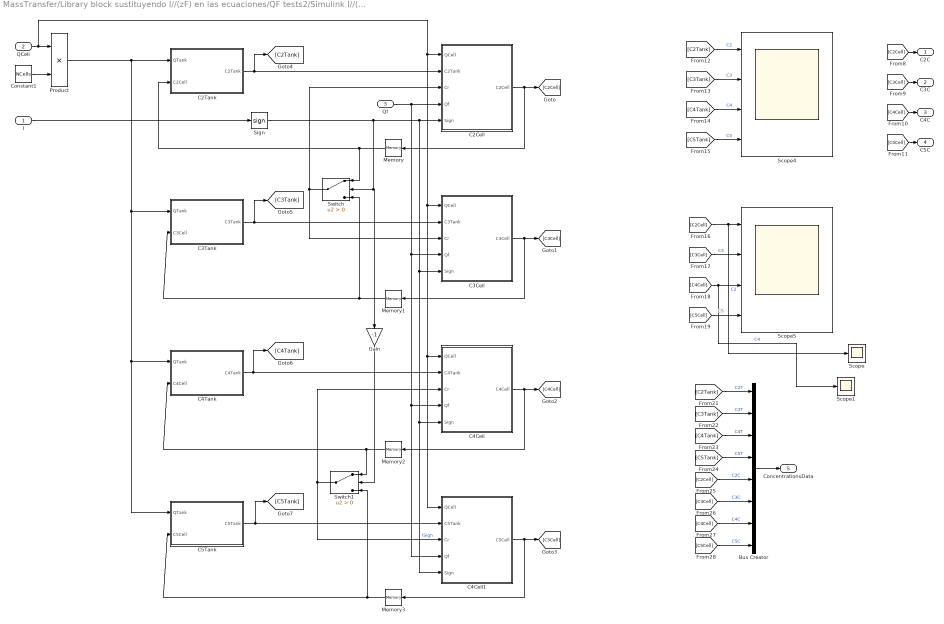
== system MassTransfer/Library block sustituyendo I//(zF) en las ecuaciones/QF tests2/Simulink I//(zf) Cambiado ==
  I : Inport
  QCell : Inport  Port=2
  Qf : Inport  Port=3
  Bus Creator : BusCreator  Inputs=8
  C2Cell : Subsystem
  C2Tank : Subsystem
  C3Cell : Subsystem
  C3Tank : Subsystem
  C4Cell : Subsystem
  C4Cell1 : Subsystem
  C4Tank : Subsystem
  C5Tank : Subsystem
  Constant1 : Constant  Value=NCells
  Gain : Gain  Gain=-1
  Memory : Memory  InitialCondition=C2Ini
  Memory1 : Memory  InitialCondition=C3Ini
  Memory2 : Memory  InitialCondition=C4Ini
  Memory3 : Memory  InitialCondition=C5Ini
  Product : Product
  Scope : Scope
  Scope1 : Scope
  Scope4 : Scope  NumInputPorts=4
  Scope5 : Scope  NumInputPorts=4
  Sign : Signum
  Switch : Switch  Criteria=u2 > Threshold  SaturateOnIntegerOverflow=off  InputSameDT=off
  Switch1 : Switch  Criteria=u2 > Threshold  SaturateOnIntegerOverflow=off  InputSameDT=off
  C2C : Outport
  C3C : Outport  Port=2
  C4C : Outport  Port=3
  C5C : Outport  Port=4
  ConcentrationsData : Outport  Port=5
  wires:
  [C5Cell] -> C5C/1
  [C3Cell] -> C3C/1
  [C2Cell] -> C2C/1
  [C4Cell] -> C4C/1
  Constant1/1 -> Product/2
  QCell/1 -> C2Cell/1(QCell), C4Cell1/1(QCell), C4Cell/1(QCell), C3Cell/1(QCell), Product/1
  [C2Tank] -> Scope4/1  "C2"
  [C3Tank] -> Scope4/2  "C3"
  [C4Tank] -> Scope4/3  "C4"
  [C5Tank] -> Scope4/4  "C5"
  [C2Cell] -> Scope/1, Scope5/1  "C2"
  [C3Cell] -> Scope5/2  "C3"
  [C4Cell] -> Scope1/1, Scope5/3  "C4"
  [C5Cell] -> Scope5/4  "C5"
  [C2Tank] -> Bus Creator/1  "C2T"
  [C3Tank] -> Bus Creator/2  "C3T"
  [C4Tank] -> Bus Creator/3  "C4T"
  [C5Tank] -> Bus Creator/4  "C5T"
  [C2Cell] -> Bus Creator/5  "C2C"
  [C3Cell] -> Bus Creator/6  "C3C"
  [C4Cell] -> Bus Creator/7  "C4C"
  [C5Cell] -> Bus Creator/8  "C5C"
  Bus Creator/1 -> ConcentrationsData/1
  Qf/1 -> C3Cell/4(Qf), C4Cell1/4(Qf), C4Cell/4(Qf), C2Cell/4(Qf)
  I/1 -> Sign/1
  Sign/1 -> Gain/1, Switch/2, C3Cell/5(Sign), C4Cell1/5(Sign), C4Cell/5(Sign), C2Cell/5(Sign)  "ISign"
  C2Tank/1(C2Tank) -> C2Cell/2(C2Tank), [C2Tank]
  C3Tank/1(C3Tank) -> [C3Tank], C3Cell/2(C3Tank)
  C4Tank/1(C4Tank) -> [C4Tank], C4Cell/2(C4Tank)
  C5Tank/1(C5Tank) -> [C5Tank], C4Cell1/2(C5Tank)
  C2Cell/1(C2Cell) -> Memory/1, [C2Cell]
  Memory/1 -> Switch/1, C2Tank/2(C2Cell)
  C3Cell/1(C3Cell) -> Memory1/1, [C3Cell]
  Memory1/1 -> Switch/3, C3Tank/2(C3Cell)
  C4Cell/1(C4Cell) -> Memory2/1, [C4Cell]
  Memory2/1 -> Switch1/1, C4Tank/2(C4Cell)
  C4Cell1/1(C5Cell) -> [C5Cell], Memory3/1
  Memory3/1 -> Switch1/3, C5Tank/2(C5Cell)
  Product/1 -> C5Tank/1(QTank), C4Tank/1(QTank), C3Tank/1(QTank), C2Tank/1(QTank)
  Switch/1 -> C3Cell/3(Cr), C2Cell/3(Cr)
  Switch1/1 -> C4Cell/3(Cr), C4Cell1/3(Cr)
  Gain/1 -> Switch1/2

== system MassTransfer/Liibrary block/Analitical/C2Cell ==
  QCell : Inport
  CTank : Inport  Port=2
  It : Inport  Port=3
  Constant : Constant  Value=-1
  Constant1 : Constant  Value=Delta
  Constant2 : Constant
  Constant3 : Constant  Value=F
  Constant4 : Constant  Value=VCell
  MATLAB Function : MATLAB Function  TreatAsAtomicUnit=on
  Memory : Memory  InitialCondition=C2Ini
  CCell : Outport
  wires:
  Constant/1 -> MATLAB Function/8(Sign)
  Constant1/1 -> MATLAB Function/9(Delta)
  Constant2/1 -> MATLAB Function/7(Z)
  QCell/1 -> MATLAB Function/1(QCell)
  Constant3/1 -> MATLAB Function/6(F)
  Constant4/1 -> MATLAB Function/4(VCell)
  MATLAB Function/1(CCell) -> Memory/1, CCell/1
  Memory/1 -> MATLAB Function/3(CCellAnt)
  It/1 -> MATLAB Function/5(It)
  CTank/1 -> MATLAB Function/2(CTank)

== system MassTransfer/Liibrary block/Analitical/C2Tank ==
  QTank : Inport
  CCell : Inport  Port=2
  Constant : Constant  Value=Delta
  Constant1 : Constant  Value=VTank
  MATLAB Function : MATLAB Function  TreatAsAtomicUnit=on
  Memory : Memory  InitialCondition=C2Ini
  Scope4 : Scope
  CTank : Outport
  wires:
  Constant/1 -> MATLAB Function/5(Delta)
  Constant1/1 -> MATLAB Function/4(VTank)
  MATLAB Function/1(CTank) -> Memory/1, CTank/1
  Memory/1 -> MATLAB Function/3(CTankAnt)
  QTank/1 -> MATLAB Function/1(Q)
  CCell/1 -> Scope4/1, MATLAB Function/2(CCell)

== system MassTransfer/Liibrary block/Analitical/C3Cell ==
  QCell : Inport
  CTank : Inport  Port=2
  It : Inport  Port=3
  Constant : Constant
  Constant1 : Constant  Value=Delta
  Constant2 : Constant
  Constant3 : Constant  Value=F
  Constant4 : Constant  Value=VCell
  MATLAB Function : MATLAB Function  TreatAsAtomicUnit=on
  Memory : Memory  InitialCondition=C3Ini
  CCell : Outport
  wires:
  It/1 -> MATLAB Function/5(It)
  Memory/1 -> MATLAB Function/3(CCellAnt)
  MATLAB Function/1(CCell) -> Memory/1, CCell/1
  Constant4/1 -> MATLAB Function/4(VCell)
  Constant3/1 -> MATLAB Function/6(F)
  QCell/1 -> MATLAB Function/1(QCell)
  Constant2/1 -> MATLAB Function/7(Z)
  Constant1/1 -> MATLAB Function/9(Delta)
  Constant/1 -> MATLAB Function/8(Sign)
  CTank/1 -> MATLAB Function/2(CTank)

== system MassTransfer/Liibrary block/Analitical/C3Tank ==
  QTank : Inport
  CCell : Inport  Port=2
  Constant : Constant  Value=Delta
  Constant1 : Constant  Value=VTank
  MATLAB Function : MATLAB Function  TreatAsAtomicUnit=on
  Memory : Memory  InitialCondition=C3Ini
  CTank : Outport
  wires:
  QTank/1 -> MATLAB Function/1(Q)
  Memory/1 -> MATLAB Function/3(CTankAnt)
  MATLAB Function/1(CTank) -> Memory/1, CTank/1
  Constant1/1 -> MATLAB Function/4(VTank)
  Constant/1 -> MATLAB Function/5(Delta)
  CCell/1 -> MATLAB Function/2(CCell)

== system MassTransfer/Liibrary block/Analitical/C4Cell ==
  QCell : Inport
  CTank : Inport  Port=2
  It : Inport  Port=3
  Constant : Constant
  Constant1 : Constant  Value=Delta
  Constant2 : Constant
  Constant3 : Constant  Value=F
  Constant4 : Constant  Value=VCell
  MATLAB Function : MATLAB Function  TreatAsAtomicUnit=on
  Memory : Memory  InitialCondition=C4Ini
  CCell : Outport
  wires:
  Constant/1 -> MATLAB Function/8(Sign)
  Constant1/1 -> MATLAB Function/9(Delta)
  Constant2/1 -> MATLAB Function/7(Z)
  QCell/1 -> MATLAB Function/1(QCell)
  Constant3/1 -> MATLAB Function/6(F)
  Constant4/1 -> MATLAB Function/4(VCell)
  MATLAB Function/1(CCell) -> Memory/1, CCell/1
  Memory/1 -> MATLAB Function/3(CCellAnt)
  It/1 -> MATLAB Function/5(It)
  CTank/1 -> MATLAB Function/2(CTank)

== system MassTransfer/Liibrary block/Analitical/C4Tank ==
  QTank : Inport
  CCell : Inport  Port=2
  Constant : Constant  Value=Delta
  Constant1 : Constant  Value=VTank
  MATLAB Function : MATLAB Function  TreatAsAtomicUnit=on
  Memory : Memory  InitialCondition=C4Ini
  CTank : Outport
  wires:
  Constant/1 -> MATLAB Function/5(Delta)
  Constant1/1 -> MATLAB Function/4(VTank)
  MATLAB Function/1(CTank) -> Memory/1, CTank/1
  Memory/1 -> MATLAB Function/3(CTankAnt)
  QTank/1 -> MATLAB Function/1(Q)
  CCell/1 -> MATLAB Function/2(CCell)

== system MassTransfer/Liibrary block/Analitical/C5Cell ==
  QCell : Inport
  CTank : Inport  Port=2
  It : Inport  Port=3
  Constant : Constant  Value=-1
  Constant1 : Constant  Value=Delta
  Constant2 : Constant
  Constant3 : Constant  Value=F
  Constant4 : Constant  Value=VCell
  MATLAB Function : MATLAB Function  TreatAsAtomicUnit=on
  Memory : Memory  InitialCondition=C5Ini
  CCell : Outport
  wires:
  It/1 -> MATLAB Function/5(It)
  Memory/1 -> MATLAB Function/3(CCellAnt)
  MATLAB Function/1(CCell) -> Memory/1, CCell/1
  Constant4/1 -> MATLAB Function/4(VCell)
  Constant3/1 -> MATLAB Function/6(F)
  QCell/1 -> MATLAB Function/1(QCell)
  Constant2/1 -> MATLAB Function/7(Z)
  Constant1/1 -> MATLAB Function/9(Delta)
  Constant/1 -> MATLAB Function/8(Sign)
  CTank/1 -> MATLAB Function/2(CTank)

== system MassTransfer/Liibrary block/Analitical/C5Tank ==
  QTank : Inport
  CCell : Inport  Port=2
  Constant : Constant  Value=Delta
  Constant1 : Constant  Value=VTank
  MATLAB Function : MATLAB Function  TreatAsAtomicUnit=on
  Memory : Memory  InitialCondition=C5Ini
  Scope : Scope
  CTank : Outport
  wires:
  QTank/1 -> MATLAB Function/1(Q)
  Memory/1 -> MATLAB Function/3(CTankAnt)
  MATLAB Function/1(CTank) -> Memory/1, CTank/1
  Constant1/1 -> MATLAB Function/4(VTank)
  Constant/1 -> MATLAB Function/5(Delta)
  CCell/1 -> MATLAB Function/2(CCell), Scope/1
